simulink model "bai1"  (R2018b)
settings: Solver=FixedStepAuto  StartTime=0.0  StopTime=0.5  FixedStep=0.00005  RelTol=1e-3
undefined symbols (not defined in the file): La, OmegaN, Ra, Td, Tf, Zeta
settings Model: Creator=User  LastModifiedBy=User

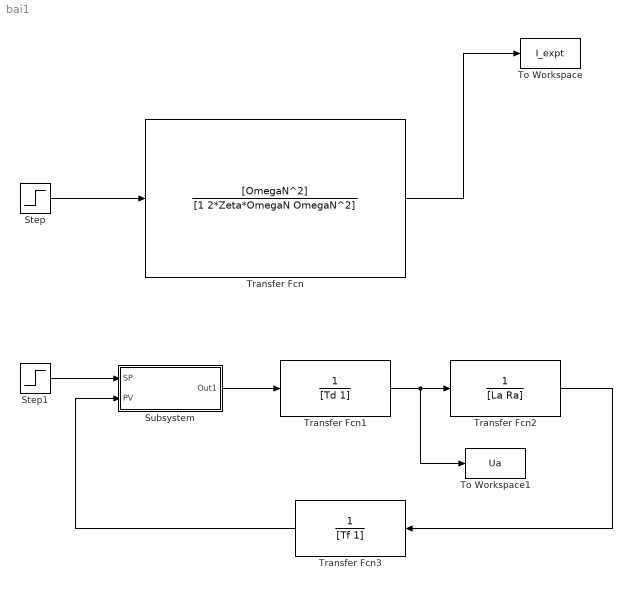
== system bai1 ==
  Step : Step  Time=0  After=62.5  SampleTime=0
  Step1 : Step  Time=0  After=62.5  SampleTime=0
  Subsystem : Subsystem
  To Workspace : ToWorkspace  VariableName=I_expt  SaveFormat=Timeseries  SampleTime=-1
  To Workspace1 : ToWorkspace  VariableName=Ua  SaveFormat=Timeseries  SampleTime=-1
  Transfer Fcn : TransferFcn  Numerator=[OmegaN^2]  Denominator=[1 2*Zeta*OmegaN OmegaN^2]
  Transfer Fcn1 : TransferFcn  Denominator=[Td 1]
  Transfer Fcn2 : TransferFcn  Denominator=[La Ra]
  Transfer Fcn3 : TransferFcn  Denominator=[Tf 1]
  wires:
  Step/1 -> Transfer Fcn/1
  Transfer Fcn/1 -> To Workspace/1
  Step1/1 -> Subsystem/1(SP)
  Subsystem/1(Out1) -> Transfer Fcn1/1
  Transfer Fcn1/1 -> To Workspace1/1, Transfer Fcn2/1
  Transfer Fcn3/1 -> Subsystem/2(PV)
  Transfer Fcn2/1 -> Transfer Fcn3/1

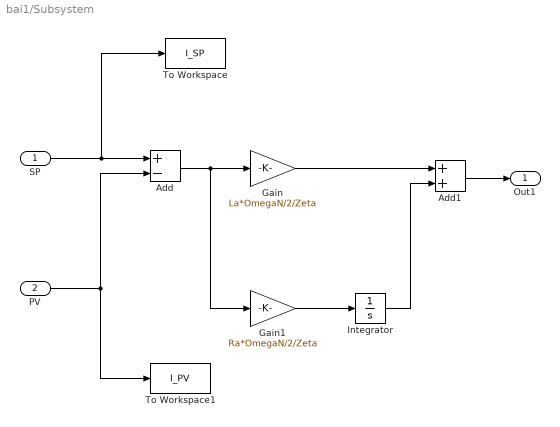
== system bai1/Subsystem ==
  SP : Inport
  PV : Inport  Port=2
  Add : Sum  Inputs=+-
  Add1 : Sum
  Gain : Gain  Gain=La*OmegaN/2/Zeta
  Gain1 : Gain  Gain=Ra*OmegaN/2/Zeta
  Integrator : Integrator
  To Workspace : ToWorkspace  VariableName=I_SP  SaveFormat=Timeseries  SampleTime=-1
  To Workspace1 : ToWorkspace  VariableName=I_PV  SaveFormat=Timeseries  SampleTime=-1
  Out1 : Outport
  wires:
  SP/1 -> To Workspace/1, Add/1
  PV/1 -> Add/2, To Workspace1/1
  Add/1 -> Gain1/1, Gain/1
  Gain1/1 -> Integrator/1
  Gain/1 -> Add1/1
  Integrator/1 -> Add1/2
  Add1/1 -> Out1/1
